simulink model "Minh_Final_project_Inverter_V3"  (R2024b)
settings: Solver=VariableStepAuto  StartTime=0.0  StopTime=100  FixedStep=1e-5  MaxStep=1e-3  MinStep=1e-8  RelTol=1e-2
values from neighbouring files (symbols this model uses):
  A_f = 1.24    [Minh_Inverter_Init.m]
  C_d = 0.7041    [Minh_Inverter_Init.m]
  C_rr = 0.02    [Minh_Inverter_Init.m]
  Current_max = min(InvCurr,mCurr)    [Minh_Inverter_Init.m]
  Encoder_Offset = (PhaseA_offset/ppair)*pi/180    (= -0.785398163397)    [Minh_Inverter_Init.m]
  g = 9.8    [Minh_Inverter_Init.m]
  J = mrot*r^2/k^2 + 0.0045    (= 0.8303048)    [Minh_Inverter_Init.m]
  k = 1    [Minh_Inverter_Init.m]
  lambda = 0.0375    [Minh_Inverter_Init.m]
  Ld = 0.1e-3    (= 0.0001)    [Minh_Inverter_Init.m]
  Lq = Ld    (= 0.0001)    [Minh_Inverter_Init.m]
  m = 1    [Minh_Inverter_Init.m]
  ppair = 4    [Minh_Inverter_Init.m]
  r = 0.4064/2    (= 0.2032)    [Minh_Inverter_Init.m]
  rho = 1.2    [Minh_Inverter_Init.m]
  Rs = (Rpp^2)/(Rpp*3)    (= 0.00433333333333)    [Minh_Inverter_Init.m]
  speed_max = rpm_max*2*pi/60    (= 523.598775598)    [Minh_Inverter_Init.m]
  Torque_max = Current_max*3*lambda*ppair/2    [Minh_Inverter_Init.m]
  Voltage_max = min(V_bat,mVolt)    [Minh_Inverter_Init.m]
undefined symbols (not defined in the file or in its folder): Down, Up
libraries: nesl_utility x27, fl_lib x23, slpidlib x12, ee_lib x11, spsabctodq0Lib x4, simulink x3, spsdq0toabcLib x2, eePwmGenerator x2, mcbresolverdecoderlib x1, eeResolverToDigitalConverter x1
(part 3 of 3)

== system Minh_Final_project_Inverter_V3/Ideal Simulation Continous Time/PWM and PMSM Simscape (real model)/Resolver1 ==
  Meas Vxy : Subsystem
  Resolver : ee_lib/Sensors & Transducers/Resolver  parameterization=1  ratio=0.5  Rr=70 Ohm  Rs=180 Ohm  Xr=100 Ohm  Xs=300 Ohm  omega=10 kHz  Lr=0.0016 H  Ls=0.0048 H  k=0.35  N=4  theta_specify=off  theta_priority=High  theta=0 deg  theta_nominal_specify=off  theta_nominal_value=1  theta_nominal_unit=deg
      settings: InternalSimscapePortConfiguration="{\"Bottom\":[],\"Left\":[{\"id\":\"p1\",\"label\":\"p1\",\"type\":\"foundation.electrical.electrical\"},{\"id\":\"p2\",\"label\":\"p2\",\"type\":\"foundation.electrical.electrical\"},{\"id\":\"R\",\"label\":\"R\",\"type\":\"foundation.mechanical.rotational.rotational\"},{\"id\":\"C\",\"label\":\"C\",\"type\":\"foundation.mechanical.rotational.rotational\"}],\"Right\":[{\"id\":\"x1\",\"label\":\"x1\",\"type\":\"foundation.electrical.electrical\"},{\"id\":\"x2\",\"label\":\"x2\",\"type\":\"foundation.electrical.electrical\"},{\"id\":\"y1\",\"label\":\"y1\",\"type\":\"foundation.electrical.electrical\"},{\"id\":\"y2\",\"label\":\"y2\",\"type\":\"foundation.electrical.electrical\"}],\"Top\":[]}"
  Resolver Decoder : mcbresolverdecoderlib/Resolver Decoder  ComputeMethod=Arithmetic  MechPos=on  TrigElecPos=off  Speed=off  Pr=1  ExcitationMethod=Sinusoidal Excitation  Normalization=off  PhaseDelay=0  SampleLength=16  Pm=ppair  RoundingMethod=Zero  BlockSampleTime=50e-6  MaximumApplicationFreq=7500  SpeedCutoffFreq=10  N_points=1024  Threshold=2e-2  PositionUnit=Radians  PositionDataType=single  SpeedUnit=Degrees/Sec  BaseSpeed=2000  SpeedDataType=single  TableDataType=single  Kp=942.4778  Ki=222066.099  Offset=0
      settings: LibrarySourceBlock=mcblib/Sensor Decoders/Resolver Decoder
  Resolver-to-Digital Converter : eeResolverToDigitalConverter/Resolver-to-Digital Converter  N=ppair  Kp=15  Ki=2.5e5  theta0=0  Ts=-1
  Scope : Scope  NumInputPorts=2
  Vp : Subsystem
  R : PMIOPort  Side=Left
  C : PMIOPort  Port=2  Side=Left
  R1 : PMIOPort  Port=3  Side=Right
  C1 : PMIOPort  Port=4  Side=Right
  wires:
  Meas Vxy/1(Vx) -> Resolver-to-Digital Converter/2
  Meas Vxy/2(Vy) -> Resolver-to-Digital Converter/3
  Vp/1(Vp) -> Resolver-to-Digital Converter/1
  Resolver-to-Digital Converter/1 -> Scope/1
  Resolver-to-Digital Converter/2 -> Scope/2
  connections:
  Resolver/LConn4 -- C/RConn1 -- C1/RConn1
  R/RConn1 -- R1/RConn1 -- Resolver/LConn3
  Meas Vxy/LConn2 -- Resolver/RConn2
  Resolver/RConn1 -- Meas Vxy/LConn1
  Meas Vxy/LConn3 -- Resolver/RConn3
  Meas Vxy/LConn4 -- Resolver/RConn4
  Vp/RConn1 -- Resolver/LConn1
  Vp/RConn2 -- Resolver/LConn2

== system Minh_Final_project_Inverter_V3/Ideal Simulation Discrete Time/FIELD ORIENTED CONTROLLER/Decoupling ==
  Iq : Inport
  Id : Inport  Port=2
  Speed : Inport  Port=3
  Add1 : Sum
  Gain1 : Gain  Gain=-Lq
  Gain3 : Gain  Gain=Ld
  Gain4 : Gain  Gain=lambda
  Product : Product
  Product1 : Product
  Ed : Outport
  Eq : Outport  Port=2
  wires:
  Product/1 -> Ed/1
  Gain3/1 -> Product1/1
  Product1/1 -> Add1/1
  Gain4/1 -> Add1/2
  Add1/1 -> Eq/1
  Speed/1 -> Gain4/1, Gain3/1, Gain1/1  "Electrical Speed w_e"
  Iq/1 -> Product/1
  Gain1/1 -> Product/2
  Id/1 -> Product1/2

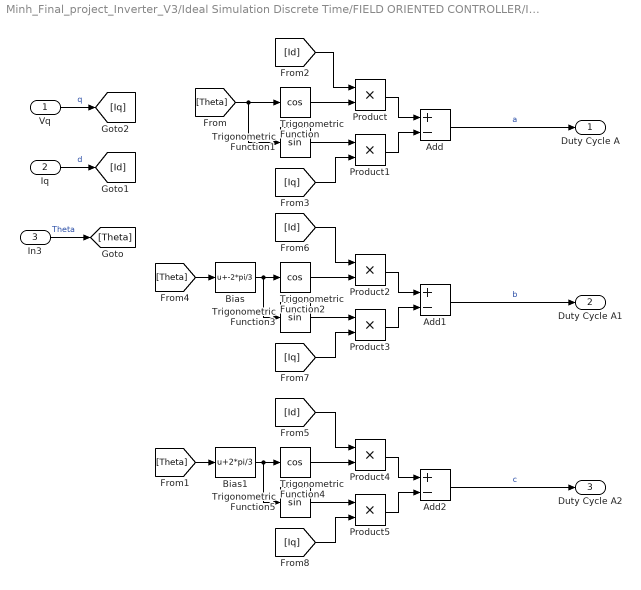
== system Minh_Final_project_Inverter_V3/Ideal Simulation Discrete Time/FIELD ORIENTED CONTROLLER/Inverse park ==
  Vq : Inport
  Iq : Inport  Port=2
  In3 : Inport  Port=3
  Add : Sum  Inputs=+-
  Add1 : Sum  Inputs=+-
  Add2 : Sum  Inputs=+-
  Bias : Bias  Bias=-2*pi/3  SaturateOnIntegerOverflow=off
  Bias1 : Bias  Bias=2*pi/3  SaturateOnIntegerOverflow=off
  Product{,1..5} (6 alike) : Product
  Trigonometric Function : Trigonometry  Operator=cos
  Trigonometric Function1 : Trigonometry
  Trigonometric Function2 : Trigonometry  Operator=cos
  Trigonometric Function3 : Trigonometry
  Trigonometric Function4 : Trigonometry  Operator=cos
  Trigonometric Function5 : Trigonometry
  Duty Cycle A : Outport
  Duty Cycle A1 : Outport  Port=2
  Duty Cycle A2 : Outport  Port=3
  wires:
  Iq/1 -> [Id]  "d"
  Vq/1 -> [Iq]  "q"
  Add/1 -> Duty Cycle A/1  "a"
  Add1/1 -> Duty Cycle A1/1  "b"
  In3/1 -> [Theta]  "Theta"
  [Theta] -> Trigonometric Function1/1, Trigonometric Function/1
  [Iq] -> Product1/2
  Trigonometric Function/1 -> Product/2
  [Id] -> Product/1
  Trigonometric Function1/1 -> Product1/1
  Product/1 -> Add/1
  Product1/1 -> Add/2
  Product3/1 -> Add1/2
  [Theta] -> Bias/1
  [Id] -> Product2/1
  Product2/1 -> Add1/1
  Trigonometric Function3/1 -> Product3/1
  [Iq] -> Product3/2
  Trigonometric Function2/1 -> Product2/2
  Bias/1 -> Trigonometric Function3/1, Trigonometric Function2/1
  Trigonometric Function4/1 -> Product4/2
  [Id] -> Product4/1
  [Theta] -> Bias1/1
  [Iq] -> Product5/2
  Add2/1 -> Duty Cycle A2/1  "c"
  Product5/1 -> Add2/2
  Trigonometric Function5/1 -> Product5/1
  Product4/1 -> Add2/1
  Bias1/1 -> Trigonometric Function5/1, Trigonometric Function4/1

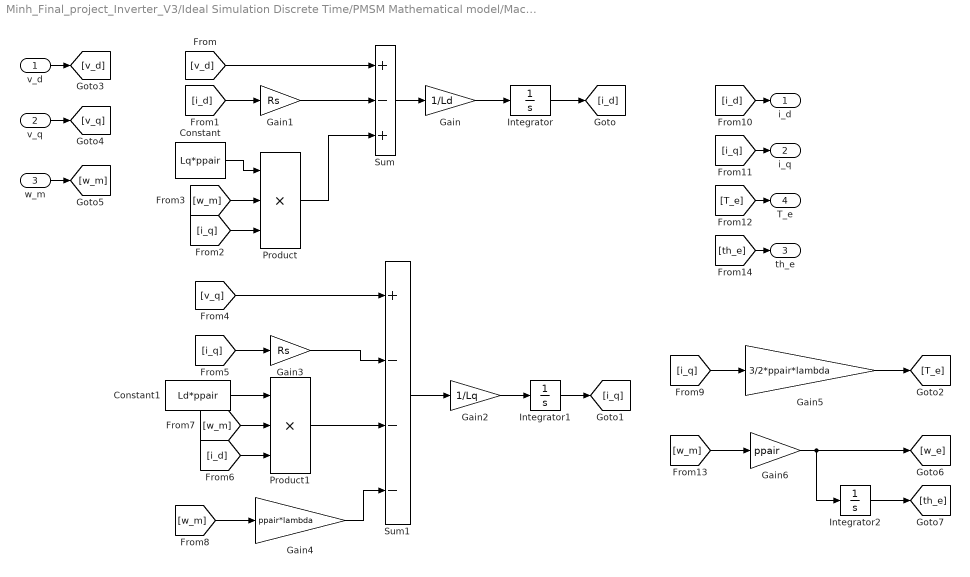
== system Minh_Final_project_Inverter_V3/Ideal Simulation Discrete Time/PMSM Mathematical model/Machine Model in DQ ==
  v_d : Inport
  v_q : Inport  Port=2
  w_m : Inport  Port=3
  Constant : Constant  Value=Lq*ppair
  Constant1 : Constant  Value=Ld*ppair
  Gain : Gain  Gain=1/Ld
  Gain1 : Gain  Gain=Rs
  Gain2 : Gain  Gain=1/Lq
  Gain3 : Gain  Gain=Rs
  Gain4 : Gain  Gain=ppair*lambda
  Gain5 : Gain  Gain=3/2*ppair*lambda
  Gain6 : Gain  Gain=ppair
  Integrator : Integrator
  Integrator1 : Integrator
  Integrator2 : Integrator
  Product : Product  Inputs=3
  Product1 : Product  Inputs=3
  Sum : Sum  Inputs=+-+
  Sum1 : Sum  Inputs=+---
  i_d : Outport
  i_q : Outport  Port=2
  th_e : Outport  Port=3
  T_e : Outport  Port=4
  wires:
  Constant/1 -> Product/1
  Product/1 -> Sum/3
  Integrator/1 -> [i_d]
  [v_d] -> Sum/1
  [w_m] -> Product1/2
  Gain4/1 -> Sum1/4
  [i_q] -> Product/3
  Sum/1 -> Gain/1
  [w_m] -> Gain4/1
  [i_d] -> Gain1/1
  Sum1/1 -> Gain2/1
  Gain/1 -> Integrator/1
  Gain5/1 -> [T_e]
  [i_q] -> Gain5/1
  Gain1/1 -> Sum/2
  Integrator1/1 -> [i_q]
  [i_q] -> Gain3/1
  Product1/1 -> Sum1/3
  Constant1/1 -> Product1/1
  Gain2/1 -> Integrator1/1
  [v_q] -> Sum1/1
  Gain3/1 -> Sum1/2
  [i_d] -> Product1/3
  [w_m] -> Product/2
  v_d/1 -> [v_d]
  v_q/1 -> [v_q]
  [i_d] -> i_d/1
  [i_q] -> i_q/1
  [T_e] -> T_e/1
  w_m/1 -> [w_m]
  [w_m] -> Gain6/1
  Gain6/1 -> Integrator2/1, [w_e]
  Integrator2/1 -> [th_e]
  [th_e] -> th_e/1

== system Minh_Final_project_Inverter_V3/Ideal Simulation Discrete Time/PMSM Mathematical model/Mechanical Model ==
  T_e : Inport
  Constant1 : Constant  Value=1/2*rho*C_d*A_f*r^2
  Constant2 : Constant  Value=m*g*C_rr
  Gain : Gain  Gain=1/k^2
  Product : Product
  Product2 : Product
  Sign : Signum
  Square : Math  Operator=square
  Subtract : Sum  Inputs=|+-
  Sum1 : Sum  Inputs=|++
  Transfer Fcn : TransferFcn  Denominator=[J 0]
  w_m : Outport
  wires:
  Constant1/1 -> Product2/1
  Transfer Fcn/1 -> Sign/1, Square/1, w_m/1
  Product2/1 -> Gain/1
  Square/1 -> Product2/2
  Subtract/1 -> Transfer Fcn/1
  T_e/1 -> Subtract/1
  Sum1/1 -> Subtract/2
  Gain/1 -> Sum1/1
  Constant2/1 -> Product/1
  Sign/1 -> Product/2
  Product/1 -> Sum1/2

== system Minh_Final_project_Inverter_V3/Ideal Simulation Discrete Time/PWM and PMSM Simscape (real model)/Gate Driver ==
  Signal : Inport
  Constant2 : Constant
  Demux3 : Demux  Outputs=3
  Demux4 : Demux  Outputs=3
  Gain2 : Gain  Gain=12
  Gain3 : Gain  Gain=12
  Scope : Scope  NumInputPorts=2
  Simulink-PS Converter{3..8} (6 alike) : nesl_utility/Simulink-PS Converter  PhysicalDomain=network_engine_domain  SubClassName=ps_input  LeftPortType=input  RightPortType=output  PseudoPeriodic=off  Frequencies=[]  NoiseDistribution=none  NoiseParameters=[]  Unit=1  AffineConversion=off  FilteringAndDerivatives=provide  SimscapeFilterOrder=1  InputFilterTimeConstant=0.001  UdotUserProvided=0
  Six-Pulse Gate Multiplexer : ee_lib/Semiconductors & Converters/Converters/Six-Pulse Gate Multiplexer  port_option=ee.enum.controlport.ps
  Subtract6 : Sum  Inputs=|+-
  Gate : PMIOPort  Side=Right
  wires:
  Subtract6/1 -> Gain2/1
  Demux3/2 -> Simulink-PS Converter6/1
  Demux4/1 -> Scope/2, Simulink-PS Converter3/1
  Gain3/1 -> Demux4/1
  Demux3/3 -> Simulink-PS Converter8/1
  Demux4/3 -> Simulink-PS Converter7/1
  Signal/1 -> Gain3/1, Subtract6/2
  Demux4/2 -> Simulink-PS Converter5/1
  Gain2/1 -> Demux3/1
  Constant2/1 -> Subtract6/1
  Demux3/1 -> Scope/1, Simulink-PS Converter4/1
  connections:
  Simulink-PS Converter8/RConn1 -- Six-Pulse Gate Multiplexer/LConn6
  Simulink-PS Converter4/RConn1 -- Six-Pulse Gate Multiplexer/LConn2
  Simulink-PS Converter7/RConn1 -- Six-Pulse Gate Multiplexer/LConn5
  Simulink-PS Converter5/RConn1 -- Six-Pulse Gate Multiplexer/LConn3
  Simulink-PS Converter3/RConn1 -- Six-Pulse Gate Multiplexer/LConn1
  Simulink-PS Converter6/RConn1 -- Six-Pulse Gate Multiplexer/LConn4
  Six-Pulse Gate Multiplexer/RConn1 -- Gate/RConn1

== system Minh_Final_project_Inverter_V3/Ideal Simulation Continous Time/PWM and PMSM Simscape (real model)/Resolver1/Meas Vxy ==
  Electrical Reference{1..4} (4 alike) : fl_lib/Electrical/Electrical Elements/Electrical Reference
  PS-Simulink Converter : nesl_utility/PS-Simulink Converter  PhysicalDomain=network_engine_domain  SubClassName=ps_output  LeftPortType=input  RightPortType=output  PseudoPeriodic=off  Frequencies=[]  VectorFormat=1-D array  Unit=1  AffineConversion=off
  PS-Simulink Converter1 : nesl_utility/PS-Simulink Converter  PhysicalDomain=network_engine_domain  SubClassName=ps_output  LeftPortType=input  RightPortType=output  PseudoPeriodic=off  Frequencies=[]  VectorFormat=1-D array  Unit=1  AffineConversion=off
  Resistor : fl_lib/Electrical/Electrical Elements/Resistor  R=1e3 Ohm  i_specify=off  i_priority=None  i=0 A  i_nominal_specify=off  i_nominal_value=1  i_nominal_unit=A  v_specify=off  v_priority=None  v=0 V  v_nominal_specify=off  v_nominal_value=1  v_nominal_unit=V
  Resistor1 : fl_lib/Electrical/Electrical Elements/Resistor  R=1e3 Ohm  i_specify=off  i_priority=None  i=0 A  i_nominal_specify=off  i_nominal_value=1  i_nominal_unit=A  v_specify=off  v_priority=None  v=0 V  v_nominal_specify=off  v_nominal_value=1  v_nominal_unit=V
  VS1 : fl_lib/Electrical/Electrical Sensors/Voltage Sensor
  VS2 : fl_lib/Electrical/Electrical Sensors/Voltage Sensor
  x1 : PMIOPort  Side=Left
  x2 : PMIOPort  Port=2  Side=Left
  y1 : PMIOPort  Port=3  Side=Left
  y2 : PMIOPort  Port=4  Side=Left
  Vx : Outport  VectorParamsAs1DForOutWhenUnconnected=off
  Vy : Outport  Port=2  VectorParamsAs1DForOutWhenUnconnected=off
  wires:
  PS-Simulink Converter/1 -> Vx/1
  PS-Simulink Converter1/1 -> Vy/1
  connections:
  VS1/LConn1 -- x1/RConn1 -- Resistor/LConn1
  VS1/RConn1 -- PS-Simulink Converter/LConn1
  Resistor/RConn1 -- x2/RConn1 -- Electrical Reference2/LConn1
  Electrical Reference1/LConn1 -- VS1/RConn2
  y2/RConn1 -- Electrical Reference4/LConn1 -- Resistor1/RConn1
  VS2/LConn1 -- y1/RConn1 -- Resistor1/LConn1
  Electrical Reference3/LConn1 -- VS2/RConn2
  VS2/RConn1 -- PS-Simulink Converter1/LConn1

== system Minh_Final_project_Inverter_V3/Ideal Simulation Continous Time/PWM and PMSM Simscape (real model)/Resolver1/Vp ==
  Electrical Reference1 : fl_lib/Electrical/Electrical Elements/Electrical Reference
  PS-Simulink Converter2 : nesl_utility/PS-Simulink Converter  PhysicalDomain=network_engine_domain  SubClassName=ps_output  LeftPortType=input  RightPortType=output  PseudoPeriodic=off  Frequencies=[]  VectorFormat=1-D array  Unit=1  AffineConversion=off
  VS1 : fl_lib/Electrical/Electrical Sensors/Voltage Sensor
  Vp1 : fl_lib/Electrical/Electrical Sources/AC Voltage Source  amp=5 V  shift=0 rad  frequency=1e4 Hz
  p1 : PMIOPort  Side=Right
  p2 : PMIOPort  Port=2  Side=Right
  Vp : Outport  VectorParamsAs1DForOutWhenUnconnected=off
  wires:
  PS-Simulink Converter2/1 -> Vp/1
  connections:
  VS1/RConn1 -- PS-Simulink Converter2/LConn1
  Electrical Reference1/LConn1 -- p2/RConn1 -- VS1/RConn2 -- Vp1/RConn1
  VS1/LConn1 -- Vp1/LConn1 -- p1/RConn1
